simulink model "TST_CoETS_TrqCalc"  (R2016b)
settings: Solver=FixedStepDiscrete  StartTime=0.0  StopTime=simTime  FixedStep=sampleTime  RelTol=1e-3
values from neighbouring files (symbols this model uses):
  testCase = 1    [initTST_CoETS_TrqCalc_001.m]    (also in initTST_CoETS_TrqCalc_002.m = 2; initTST_CoETS_TrqCalc_003.m = 3)
libraries: simulink x52, UnitTest_Lib x48
(part 2 of 2)

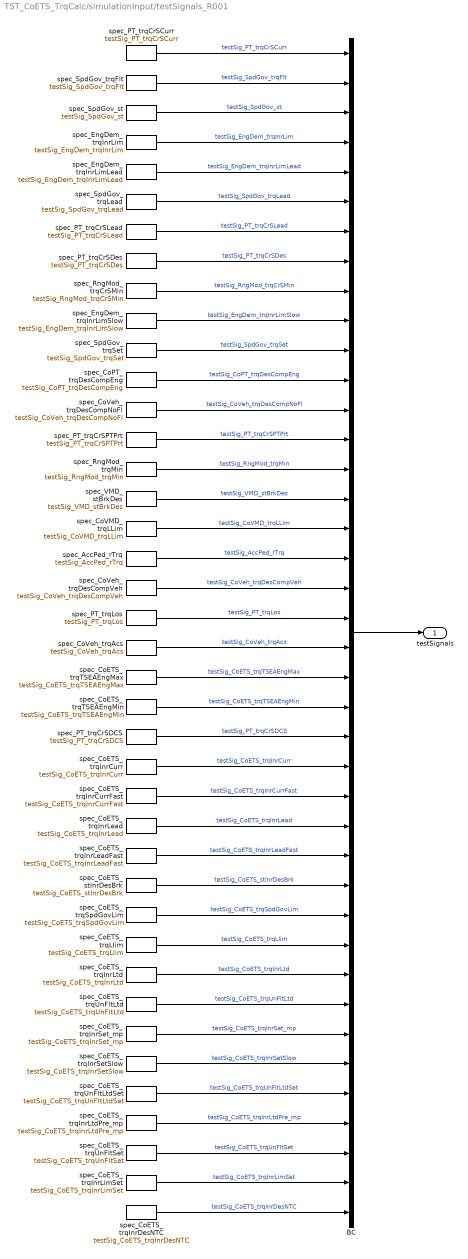
== system TST_CoETS_TrqCalc/simulationInput/testSignals_R001 ==
  BC : BusCreator  Inputs=40
  spec_AccPed_rTrq : FromWorkspace  VariableName=testSig_AccPed_rTrq  Interpolate=off  OutputAfterFinalValue=Holding final value
  spec_CoETS_stInrDesBrk : FromWorkspace  VariableName=testSig_CoETS_stInrDesBrk  Interpolate=off  OutputAfterFinalValue=Holding final value
  spec_CoETS_trqInrCurr : FromWorkspace  VariableName=testSig_CoETS_trqInrCurr  Interpolate=off  OutputAfterFinalValue=Holding final value
  spec_CoETS_trqInrCurrFast : FromWorkspace  VariableName=testSig_CoETS_trqInrCurrFast  Interpolate=off  OutputAfterFinalValue=Holding final value
  spec_CoETS_trqInrDesNTC : FromWorkspace  VariableName=testSig_CoETS_trqInrDesNTC  Interpolate=off  OutputAfterFinalValue=Holding final value
  spec_CoETS_trqInrLead : FromWorkspace  VariableName=testSig_CoETS_trqInrLead  Interpolate=off  OutputAfterFinalValue=Holding final value
  spec_CoETS_trqInrLeadFast : FromWorkspace  VariableName=testSig_CoETS_trqInrLeadFast  Interpolate=off  OutputAfterFinalValue=Holding final value
  spec_CoETS_trqInrLimSet : FromWorkspace  VariableName=testSig_CoETS_trqInrLimSet  Interpolate=off  OutputAfterFinalValue=Holding final value
  spec_CoETS_trqInrLtd : FromWorkspace  VariableName=testSig_CoETS_trqInrLtd  Interpolate=off  OutputAfterFinalValue=Holding final value
  spec_CoETS_trqInrLtdPre_mp : FromWorkspace  VariableName=testSig_CoETS_trqInrLtdPre_mp  Interpolate=off  OutputAfterFinalValue=Holding final value
  spec_CoETS_trqInrSetSlow : FromWorkspace  VariableName=testSig_CoETS_trqInrSetSlow  Interpolate=off  OutputAfterFinalValue=Holding final value
  spec_CoETS_trqInrSet_mp : FromWorkspace  VariableName=testSig_CoETS_trqInrSet_mp  Interpolate=off  OutputAfterFinalValue=Holding final value
  spec_CoETS_trqLlim : FromWorkspace  VariableName=testSig_CoETS_trqLlim  Interpolate=off  OutputAfterFinalValue=Holding final value
  spec_CoETS_trqSpdGovLim : FromWorkspace  VariableName=testSig_CoETS_trqSpdGovLim  Interpolate=off  OutputAfterFinalValue=Holding final value
  spec_CoETS_trqTSEAEngMax : FromWorkspace  VariableName=testSig_CoETS_trqTSEAEngMax  Interpolate=off  OutputAfterFinalValue=Holding final value
  spec_CoETS_trqTSEAEngMin : FromWorkspace  VariableName=testSig_CoETS_trqTSEAEngMin  Interpolate=off  OutputAfterFinalValue=Holding final value
  spec_CoETS_trqUnFltLtd : FromWorkspace  VariableName=testSig_CoETS_trqUnFltLtd  Interpolate=off  OutputAfterFinalValue=Holding final value
  spec_CoETS_trqUnFltLtdSet : FromWorkspace  VariableName=testSig_CoETS_trqUnFltLtdSet  Interpolate=off  OutputAfterFinalValue=Holding final value
  spec_CoETS_trqUnFltSet : FromWorkspace  VariableName=testSig_CoETS_trqUnFltSet  Interpolate=off  OutputAfterFinalValue=Holding final value
  spec_CoPT_trqDesCompEng : FromWorkspace  VariableName=testSig_CoPT_trqDesCompEng  Interpolate=off  OutputAfterFinalValue=Holding final value
  spec_CoVMD_trqLLim : FromWorkspace  VariableName=testSig_CoVMD_trqLLim  Interpolate=off  OutputAfterFinalValue=Holding final value
  spec_CoVeh_trqAcs : FromWorkspace  VariableName=testSig_CoVeh_trqAcs  Interpolate=off  OutputAfterFinalValue=Holding final value
  spec_CoVeh_trqDesCompNoFl : FromWorkspace  VariableName=testSig_CoVeh_trqDesCompNoFl  Interpolate=off  OutputAfterFinalValue=Holding final value
  spec_CoVeh_trqDesCompVeh : FromWorkspace  VariableName=testSig_CoVeh_trqDesCompVeh  Interpolate=off  OutputAfterFinalValue=Holding final value
  spec_EngDem_trqInrLim : FromWorkspace  VariableName=testSig_EngDem_trqInrLim  Interpolate=off  OutputAfterFinalValue=Holding final value
  spec_EngDem_trqInrLimLead : FromWorkspace  VariableName=testSig_EngDem_trqInrLimLead  Interpolate=off  OutputAfterFinalValue=Holding final value
  spec_EngDem_trqInrLimSlow : FromWorkspace  VariableName=testSig_EngDem_trqInrLimSlow  Interpolate=off  OutputAfterFinalValue=Holding final value
  spec_PT_trqCrSCurr : FromWorkspace  VariableName=testSig_PT_trqCrSCurr  Interpolate=off  OutputAfterFinalValue=Holding final value
  spec_PT_trqCrSDCS : FromWorkspace  VariableName=testSig_PT_trqCrSDCS  Interpolate=off  OutputAfterFinalValue=Holding final value
  spec_PT_trqCrSDes : FromWorkspace  VariableName=testSig_PT_trqCrSDes  Interpolate=off  OutputAfterFinalValue=Holding final value
  spec_PT_trqCrSLead : FromWorkspace  VariableName=testSig_PT_trqCrSLead  Interpolate=off  OutputAfterFinalValue=Holding final value
  spec_PT_trqCrSPTPrt : FromWorkspace  VariableName=testSig_PT_trqCrSPTPrt  Interpolate=off  OutputAfterFinalValue=Holding final value
  spec_PT_trqLos : FromWorkspace  VariableName=testSig_PT_trqLos  Interpolate=off  OutputAfterFinalValue=Holding final value
  spec_RngMod_trqCrSMin : FromWorkspace  VariableName=testSig_RngMod_trqCrSMin  Interpolate=off  OutputAfterFinalValue=Holding final value
  spec_RngMod_trqMin : FromWorkspace  VariableName=testSig_RngMod_trqMin  Interpolate=off  OutputAfterFinalValue=Holding final value
  spec_SpdGov_st : FromWorkspace  VariableName=testSig_SpdGov_st  Interpolate=off  OutputAfterFinalValue=Holding final value
  spec_SpdGov_trqFlt : FromWorkspace  VariableName=testSig_SpdGov_trqFlt  Interpolate=off  OutputAfterFinalValue=Holding final value
  spec_SpdGov_trqLead : FromWorkspace  VariableName=testSig_SpdGov_trqLead  Interpolate=off  OutputAfterFinalValue=Holding final value
  spec_SpdGov_trqSet : FromWorkspace  VariableName=testSig_SpdGov_trqSet  Interpolate=off  OutputAfterFinalValue=Holding final value
  spec_VMD_stBrkDes : FromWorkspace  VariableName=testSig_VMD_stBrkDes  Interpolate=off  OutputAfterFinalValue=Holding final value
  testSignals : Outport
  wires:
  BC/1 -> testSignals/1
  spec_PT_trqCrSCurr/1 -> BC/1  "testSig_PT_trqCrSCurr"
  spec_SpdGov_trqFlt/1 -> BC/2  "testSig_SpdGov_trqFlt"
  spec_SpdGov_st/1 -> BC/3  "testSig_SpdGov_st"
  spec_EngDem_trqInrLim/1 -> BC/4  "testSig_EngDem_trqInrLim"
  spec_EngDem_trqInrLimLead/1 -> BC/5  "testSig_EngDem_trqInrLimLead"
  spec_SpdGov_trqLead/1 -> BC/6  "testSig_SpdGov_trqLead"
  spec_PT_trqCrSLead/1 -> BC/7  "testSig_PT_trqCrSLead"
  spec_PT_trqCrSDes/1 -> BC/8  "testSig_PT_trqCrSDes"
  spec_RngMod_trqCrSMin/1 -> BC/9  "testSig_RngMod_trqCrSMin"
  spec_EngDem_trqInrLimSlow/1 -> BC/10  "testSig_EngDem_trqInrLimSlow"
  spec_SpdGov_trqSet/1 -> BC/11  "testSig_SpdGov_trqSet"
  spec_CoPT_trqDesCompEng/1 -> BC/12  "testSig_CoPT_trqDesCompEng"
  spec_CoVeh_trqDesCompNoFl/1 -> BC/13  "testSig_CoVeh_trqDesCompNoFl"
  spec_PT_trqCrSPTPrt/1 -> BC/14  "testSig_PT_trqCrSPTPrt"
  spec_RngMod_trqMin/1 -> BC/15  "testSig_RngMod_trqMin"
  spec_VMD_stBrkDes/1 -> BC/16  "testSig_VMD_stBrkDes"
  spec_CoVMD_trqLLim/1 -> BC/17  "testSig_CoVMD_trqLLim"
  spec_AccPed_rTrq/1 -> BC/18  "testSig_AccPed_rTrq"
  spec_CoVeh_trqDesCompVeh/1 -> BC/19  "testSig_CoVeh_trqDesCompVeh"
  spec_PT_trqLos/1 -> BC/20  "testSig_PT_trqLos"
  spec_CoVeh_trqAcs/1 -> BC/21  "testSig_CoVeh_trqAcs"
  spec_CoETS_trqTSEAEngMax/1 -> BC/22  "testSig_CoETS_trqTSEAEngMax"
  spec_CoETS_trqTSEAEngMin/1 -> BC/23  "testSig_CoETS_trqTSEAEngMin"
  spec_PT_trqCrSDCS/1 -> BC/24  "testSig_PT_trqCrSDCS"
  spec_CoETS_trqInrCurr/1 -> BC/25  "testSig_CoETS_trqInrCurr"
  spec_CoETS_trqInrCurrFast/1 -> BC/26  "testSig_CoETS_trqInrCurrFast"
  spec_CoETS_trqInrLead/1 -> BC/27  "testSig_CoETS_trqInrLead"
  spec_CoETS_trqInrLeadFast/1 -> BC/28  "testSig_CoETS_trqInrLeadFast"
  spec_CoETS_stInrDesBrk/1 -> BC/29  "testSig_CoETS_stInrDesBrk"
  spec_CoETS_trqSpdGovLim/1 -> BC/30  "testSig_CoETS_trqSpdGovLim"
  spec_CoETS_trqLlim/1 -> BC/31  "testSig_CoETS_trqLlim"
  spec_CoETS_trqInrLtd/1 -> BC/32  "testSig_CoETS_trqInrLtd"
  spec_CoETS_trqUnFltLtd/1 -> BC/33  "testSig_CoETS_trqUnFltLtd"
  spec_CoETS_trqInrSet_mp/1 -> BC/34  "testSig_CoETS_trqInrSet_mp"
  spec_CoETS_trqInrSetSlow/1 -> BC/35  "testSig_CoETS_trqInrSetSlow"
  spec_CoETS_trqUnFltLtdSet/1 -> BC/36  "testSig_CoETS_trqUnFltLtdSet"
  spec_CoETS_trqInrLtdPre_mp/1 -> BC/37  "testSig_CoETS_trqInrLtdPre_mp"
  spec_CoETS_trqUnFltSet/1 -> BC/38  "testSig_CoETS_trqUnFltSet"
  spec_CoETS_trqInrLimSet/1 -> BC/39  "testSig_CoETS_trqInrLimSet"
  spec_CoETS_trqInrDesNTC/1 -> BC/40  "testSig_CoETS_trqInrDesNTC"

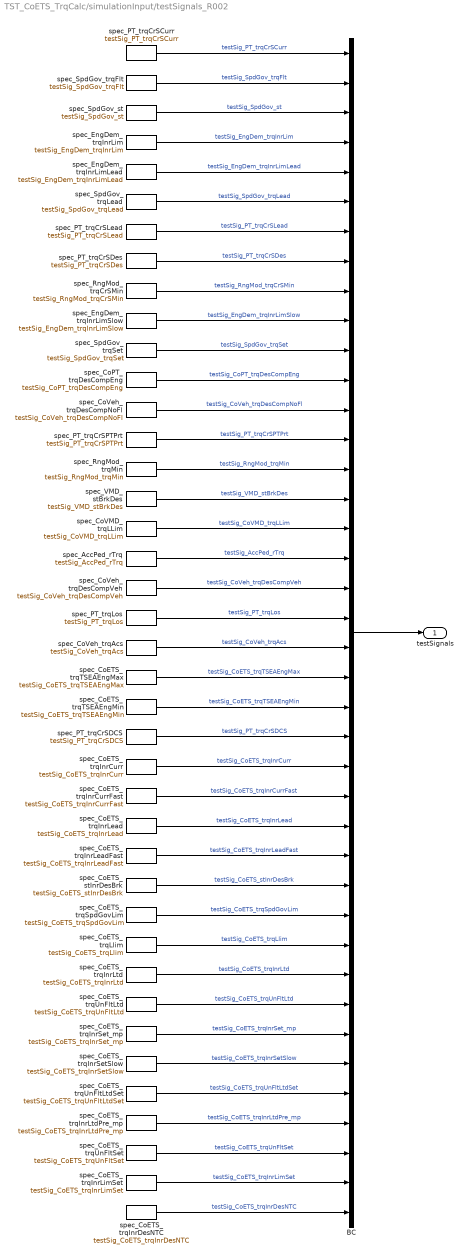
== system TST_CoETS_TrqCalc/simulationInput/testSignals_R002 ==
  BC : BusCreator  Inputs=40
  spec_AccPed_rTrq : FromWorkspace  VariableName=testSig_AccPed_rTrq  Interpolate=off  OutputAfterFinalValue=Holding final value
  spec_CoETS_stInrDesBrk : FromWorkspace  VariableName=testSig_CoETS_stInrDesBrk  Interpolate=off  OutputAfterFinalValue=Holding final value
  spec_CoETS_trqInrCurr : FromWorkspace  VariableName=testSig_CoETS_trqInrCurr  Interpolate=off  OutputAfterFinalValue=Holding final value
  spec_CoETS_trqInrCurrFast : FromWorkspace  VariableName=testSig_CoETS_trqInrCurrFast  Interpolate=off  OutputAfterFinalValue=Holding final value
  spec_CoETS_trqInrDesNTC : FromWorkspace  VariableName=testSig_CoETS_trqInrDesNTC  Interpolate=off  OutputAfterFinalValue=Holding final value
  spec_CoETS_trqInrLead : FromWorkspace  VariableName=testSig_CoETS_trqInrLead  Interpolate=off  OutputAfterFinalValue=Holding final value
  spec_CoETS_trqInrLeadFast : FromWorkspace  VariableName=testSig_CoETS_trqInrLeadFast  Interpolate=off  OutputAfterFinalValue=Holding final value
  spec_CoETS_trqInrLimSet : FromWorkspace  VariableName=testSig_CoETS_trqInrLimSet  Interpolate=off  OutputAfterFinalValue=Holding final value
  spec_CoETS_trqInrLtd : FromWorkspace  VariableName=testSig_CoETS_trqInrLtd  Interpolate=off  OutputAfterFinalValue=Holding final value
  spec_CoETS_trqInrLtdPre_mp : FromWorkspace  VariableName=testSig_CoETS_trqInrLtdPre_mp  Interpolate=off  OutputAfterFinalValue=Holding final value
  spec_CoETS_trqInrSetSlow : FromWorkspace  VariableName=testSig_CoETS_trqInrSetSlow  Interpolate=off  OutputAfterFinalValue=Holding final value
  spec_CoETS_trqInrSet_mp : FromWorkspace  VariableName=testSig_CoETS_trqInrSet_mp  Interpolate=off  OutputAfterFinalValue=Holding final value
  spec_CoETS_trqLlim : FromWorkspace  VariableName=testSig_CoETS_trqLlim  Interpolate=off  OutputAfterFinalValue=Holding final value
  spec_CoETS_trqSpdGovLim : FromWorkspace  VariableName=testSig_CoETS_trqSpdGovLim  Interpolate=off  OutputAfterFinalValue=Holding final value
  spec_CoETS_trqTSEAEngMax : FromWorkspace  VariableName=testSig_CoETS_trqTSEAEngMax  Interpolate=off  OutputAfterFinalValue=Holding final value
  spec_CoETS_trqTSEAEngMin : FromWorkspace  VariableName=testSig_CoETS_trqTSEAEngMin  Interpolate=off  OutputAfterFinalValue=Holding final value
  spec_CoETS_trqUnFltLtd : FromWorkspace  VariableName=testSig_CoETS_trqUnFltLtd  Interpolate=off  OutputAfterFinalValue=Holding final value
  spec_CoETS_trqUnFltLtdSet : FromWorkspace  VariableName=testSig_CoETS_trqUnFltLtdSet  Interpolate=off  OutputAfterFinalValue=Holding final value
  spec_CoETS_trqUnFltSet : FromWorkspace  VariableName=testSig_CoETS_trqUnFltSet  Interpolate=off  OutputAfterFinalValue=Holding final value
  spec_CoPT_trqDesCompEng : FromWorkspace  VariableName=testSig_CoPT_trqDesCompEng  Interpolate=off  OutputAfterFinalValue=Holding final value
  spec_CoVMD_trqLLim : FromWorkspace  VariableName=testSig_CoVMD_trqLLim  Interpolate=off  OutputAfterFinalValue=Holding final value
  spec_CoVeh_trqAcs : FromWorkspace  VariableName=testSig_CoVeh_trqAcs  Interpolate=off  OutputAfterFinalValue=Holding final value
  spec_CoVeh_trqDesCompNoFl : FromWorkspace  VariableName=testSig_CoVeh_trqDesCompNoFl  Interpolate=off  OutputAfterFinalValue=Holding final value
  spec_CoVeh_trqDesCompVeh : FromWorkspace  VariableName=testSig_CoVeh_trqDesCompVeh  Interpolate=off  OutputAfterFinalValue=Holding final value
  spec_EngDem_trqInrLim : FromWorkspace  VariableName=testSig_EngDem_trqInrLim  Interpolate=off  OutputAfterFinalValue=Holding final value
  spec_EngDem_trqInrLimLead : FromWorkspace  VariableName=testSig_EngDem_trqInrLimLead  Interpolate=off  OutputAfterFinalValue=Holding final value
  spec_EngDem_trqInrLimSlow : FromWorkspace  VariableName=testSig_EngDem_trqInrLimSlow  Interpolate=off  OutputAfterFinalValue=Holding final value
  spec_PT_trqCrSCurr : FromWorkspace  VariableName=testSig_PT_trqCrSCurr  Interpolate=off  OutputAfterFinalValue=Holding final value
  spec_PT_trqCrSDCS : FromWorkspace  VariableName=testSig_PT_trqCrSDCS  Interpolate=off  OutputAfterFinalValue=Holding final value
  spec_PT_trqCrSDes : FromWorkspace  VariableName=testSig_PT_trqCrSDes  Interpolate=off  OutputAfterFinalValue=Holding final value
  spec_PT_trqCrSLead : FromWorkspace  VariableName=testSig_PT_trqCrSLead  Interpolate=off  OutputAfterFinalValue=Holding final value
  spec_PT_trqCrSPTPrt : FromWorkspace  VariableName=testSig_PT_trqCrSPTPrt  Interpolate=off  OutputAfterFinalValue=Holding final value
  spec_PT_trqLos : FromWorkspace  VariableName=testSig_PT_trqLos  Interpolate=off  OutputAfterFinalValue=Holding final value
  spec_RngMod_trqCrSMin : FromWorkspace  VariableName=testSig_RngMod_trqCrSMin  Interpolate=off  OutputAfterFinalValue=Holding final value
  spec_RngMod_trqMin : FromWorkspace  VariableName=testSig_RngMod_trqMin  Interpolate=off  OutputAfterFinalValue=Holding final value
  spec_SpdGov_st : FromWorkspace  VariableName=testSig_SpdGov_st  Interpolate=off  OutputAfterFinalValue=Holding final value
  spec_SpdGov_trqFlt : FromWorkspace  VariableName=testSig_SpdGov_trqFlt  Interpolate=off  OutputAfterFinalValue=Holding final value
  spec_SpdGov_trqLead : FromWorkspace  VariableName=testSig_SpdGov_trqLead  Interpolate=off  OutputAfterFinalValue=Holding final value
  spec_SpdGov_trqSet : FromWorkspace  VariableName=testSig_SpdGov_trqSet  Interpolate=off  OutputAfterFinalValue=Holding final value
  spec_VMD_stBrkDes : FromWorkspace  VariableName=testSig_VMD_stBrkDes  Interpolate=off  OutputAfterFinalValue=Holding final value
  testSignals : Outport
  wires:
  BC/1 -> testSignals/1
  spec_PT_trqCrSCurr/1 -> BC/1  "testSig_PT_trqCrSCurr"
  spec_SpdGov_trqFlt/1 -> BC/2  "testSig_SpdGov_trqFlt"
  spec_SpdGov_st/1 -> BC/3  "testSig_SpdGov_st"
  spec_EngDem_trqInrLim/1 -> BC/4  "testSig_EngDem_trqInrLim"
  spec_EngDem_trqInrLimLead/1 -> BC/5  "testSig_EngDem_trqInrLimLead"
  spec_SpdGov_trqLead/1 -> BC/6  "testSig_SpdGov_trqLead"
  spec_PT_trqCrSLead/1 -> BC/7  "testSig_PT_trqCrSLead"
  spec_PT_trqCrSDes/1 -> BC/8  "testSig_PT_trqCrSDes"
  spec_RngMod_trqCrSMin/1 -> BC/9  "testSig_RngMod_trqCrSMin"
  spec_EngDem_trqInrLimSlow/1 -> BC/10  "testSig_EngDem_trqInrLimSlow"
  spec_SpdGov_trqSet/1 -> BC/11  "testSig_SpdGov_trqSet"
  spec_CoPT_trqDesCompEng/1 -> BC/12  "testSig_CoPT_trqDesCompEng"
  spec_CoVeh_trqDesCompNoFl/1 -> BC/13  "testSig_CoVeh_trqDesCompNoFl"
  spec_PT_trqCrSPTPrt/1 -> BC/14  "testSig_PT_trqCrSPTPrt"
  spec_RngMod_trqMin/1 -> BC/15  "testSig_RngMod_trqMin"
  spec_VMD_stBrkDes/1 -> BC/16  "testSig_VMD_stBrkDes"
  spec_CoVMD_trqLLim/1 -> BC/17  "testSig_CoVMD_trqLLim"
  spec_AccPed_rTrq/1 -> BC/18  "testSig_AccPed_rTrq"
  spec_CoVeh_trqDesCompVeh/1 -> BC/19  "testSig_CoVeh_trqDesCompVeh"
  spec_PT_trqLos/1 -> BC/20  "testSig_PT_trqLos"
  spec_CoVeh_trqAcs/1 -> BC/21  "testSig_CoVeh_trqAcs"
  spec_CoETS_trqTSEAEngMax/1 -> BC/22  "testSig_CoETS_trqTSEAEngMax"
  spec_CoETS_trqTSEAEngMin/1 -> BC/23  "testSig_CoETS_trqTSEAEngMin"
  spec_PT_trqCrSDCS/1 -> BC/24  "testSig_PT_trqCrSDCS"
  spec_CoETS_trqInrCurr/1 -> BC/25  "testSig_CoETS_trqInrCurr"
  spec_CoETS_trqInrCurrFast/1 -> BC/26  "testSig_CoETS_trqInrCurrFast"
  spec_CoETS_trqInrLead/1 -> BC/27  "testSig_CoETS_trqInrLead"
  spec_CoETS_trqInrLeadFast/1 -> BC/28  "testSig_CoETS_trqInrLeadFast"
  spec_CoETS_stInrDesBrk/1 -> BC/29  "testSig_CoETS_stInrDesBrk"
  spec_CoETS_trqSpdGovLim/1 -> BC/30  "testSig_CoETS_trqSpdGovLim"
  spec_CoETS_trqLlim/1 -> BC/31  "testSig_CoETS_trqLlim"
  spec_CoETS_trqInrLtd/1 -> BC/32  "testSig_CoETS_trqInrLtd"
  spec_CoETS_trqUnFltLtd/1 -> BC/33  "testSig_CoETS_trqUnFltLtd"
  spec_CoETS_trqInrSet_mp/1 -> BC/34  "testSig_CoETS_trqInrSet_mp"
  spec_CoETS_trqInrSetSlow/1 -> BC/35  "testSig_CoETS_trqInrSetSlow"
  spec_CoETS_trqUnFltLtdSet/1 -> BC/36  "testSig_CoETS_trqUnFltLtdSet"
  spec_CoETS_trqInrLtdPre_mp/1 -> BC/37  "testSig_CoETS_trqInrLtdPre_mp"
  spec_CoETS_trqUnFltSet/1 -> BC/38  "testSig_CoETS_trqUnFltSet"
  spec_CoETS_trqInrLimSet/1 -> BC/39  "testSig_CoETS_trqInrLimSet"
  spec_CoETS_trqInrDesNTC/1 -> BC/40  "testSig_CoETS_trqInrDesNTC"

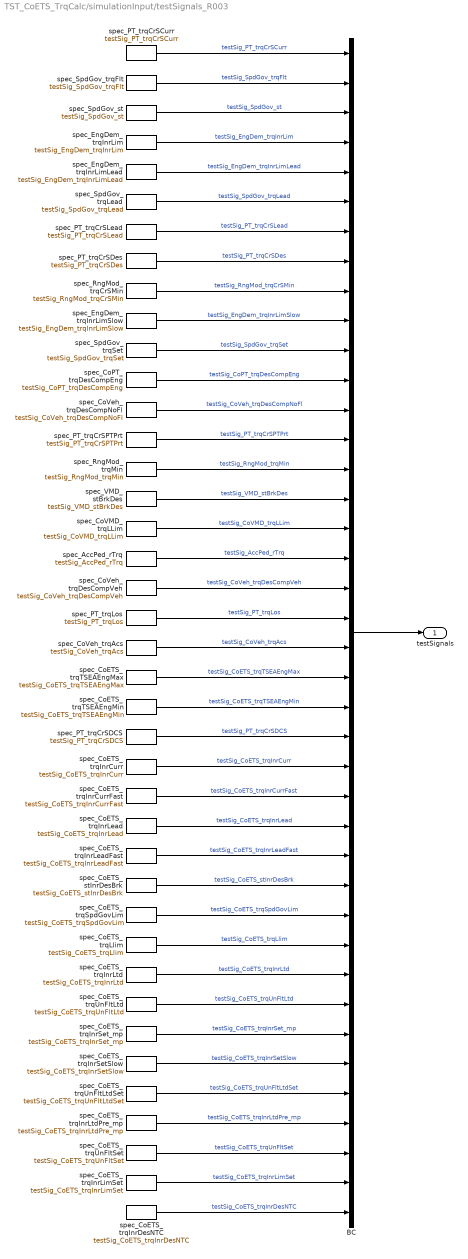
== system TST_CoETS_TrqCalc/simulationInput/testSignals_R003 ==
  BC : BusCreator  Inputs=40
  spec_AccPed_rTrq : FromWorkspace  VariableName=testSig_AccPed_rTrq  Interpolate=off  OutputAfterFinalValue=Holding final value
  spec_CoETS_stInrDesBrk : FromWorkspace  VariableName=testSig_CoETS_stInrDesBrk  Interpolate=off  OutputAfterFinalValue=Holding final value
  spec_CoETS_trqInrCurr : FromWorkspace  VariableName=testSig_CoETS_trqInrCurr  Interpolate=off  OutputAfterFinalValue=Holding final value
  spec_CoETS_trqInrCurrFast : FromWorkspace  VariableName=testSig_CoETS_trqInrCurrFast  Interpolate=off  OutputAfterFinalValue=Holding final value
  spec_CoETS_trqInrDesNTC : FromWorkspace  VariableName=testSig_CoETS_trqInrDesNTC  Interpolate=off  OutputAfterFinalValue=Holding final value
  spec_CoETS_trqInrLead : FromWorkspace  VariableName=testSig_CoETS_trqInrLead  Interpolate=off  OutputAfterFinalValue=Holding final value
  spec_CoETS_trqInrLeadFast : FromWorkspace  VariableName=testSig_CoETS_trqInrLeadFast  Interpolate=off  OutputAfterFinalValue=Holding final value
  spec_CoETS_trqInrLimSet : FromWorkspace  VariableName=testSig_CoETS_trqInrLimSet  Interpolate=off  OutputAfterFinalValue=Holding final value
  spec_CoETS_trqInrLtd : FromWorkspace  VariableName=testSig_CoETS_trqInrLtd  Interpolate=off  OutputAfterFinalValue=Holding final value
  spec_CoETS_trqInrLtdPre_mp : FromWorkspace  VariableName=testSig_CoETS_trqInrLtdPre_mp  Interpolate=off  OutputAfterFinalValue=Holding final value
  spec_CoETS_trqInrSetSlow : FromWorkspace  VariableName=testSig_CoETS_trqInrSetSlow  Interpolate=off  OutputAfterFinalValue=Holding final value
  spec_CoETS_trqInrSet_mp : FromWorkspace  VariableName=testSig_CoETS_trqInrSet_mp  Interpolate=off  OutputAfterFinalValue=Holding final value
  spec_CoETS_trqLlim : FromWorkspace  VariableName=testSig_CoETS_trqLlim  Interpolate=off  OutputAfterFinalValue=Holding final value
  spec_CoETS_trqSpdGovLim : FromWorkspace  VariableName=testSig_CoETS_trqSpdGovLim  Interpolate=off  OutputAfterFinalValue=Holding final value
  spec_CoETS_trqTSEAEngMax : FromWorkspace  VariableName=testSig_CoETS_trqTSEAEngMax  Interpolate=off  OutputAfterFinalValue=Holding final value
  spec_CoETS_trqTSEAEngMin : FromWorkspace  VariableName=testSig_CoETS_trqTSEAEngMin  Interpolate=off  OutputAfterFinalValue=Holding final value
  spec_CoETS_trqUnFltLtd : FromWorkspace  VariableName=testSig_CoETS_trqUnFltLtd  Interpolate=off  OutputAfterFinalValue=Holding final value
  spec_CoETS_trqUnFltLtdSet : FromWorkspace  VariableName=testSig_CoETS_trqUnFltLtdSet  Interpolate=off  OutputAfterFinalValue=Holding final value
  spec_CoETS_trqUnFltSet : FromWorkspace  VariableName=testSig_CoETS_trqUnFltSet  Interpolate=off  OutputAfterFinalValue=Holding final value
  spec_CoPT_trqDesCompEng : FromWorkspace  VariableName=testSig_CoPT_trqDesCompEng  Interpolate=off  OutputAfterFinalValue=Holding final value
  spec_CoVMD_trqLLim : FromWorkspace  VariableName=testSig_CoVMD_trqLLim  Interpolate=off  OutputAfterFinalValue=Holding final value
  spec_CoVeh_trqAcs : FromWorkspace  VariableName=testSig_CoVeh_trqAcs  Interpolate=off  OutputAfterFinalValue=Holding final value
  spec_CoVeh_trqDesCompNoFl : FromWorkspace  VariableName=testSig_CoVeh_trqDesCompNoFl  Interpolate=off  OutputAfterFinalValue=Holding final value
  spec_CoVeh_trqDesCompVeh : FromWorkspace  VariableName=testSig_CoVeh_trqDesCompVeh  Interpolate=off  OutputAfterFinalValue=Holding final value
  spec_EngDem_trqInrLim : FromWorkspace  VariableName=testSig_EngDem_trqInrLim  Interpolate=off  OutputAfterFinalValue=Holding final value
  spec_EngDem_trqInrLimLead : FromWorkspace  VariableName=testSig_EngDem_trqInrLimLead  Interpolate=off  OutputAfterFinalValue=Holding final value
  spec_EngDem_trqInrLimSlow : FromWorkspace  VariableName=testSig_EngDem_trqInrLimSlow  Interpolate=off  OutputAfterFinalValue=Holding final value
  spec_PT_trqCrSCurr : FromWorkspace  VariableName=testSig_PT_trqCrSCurr  Interpolate=off  OutputAfterFinalValue=Holding final value
  spec_PT_trqCrSDCS : FromWorkspace  VariableName=testSig_PT_trqCrSDCS  Interpolate=off  OutputAfterFinalValue=Holding final value
  spec_PT_trqCrSDes : FromWorkspace  VariableName=testSig_PT_trqCrSDes  Interpolate=off  OutputAfterFinalValue=Holding final value
  spec_PT_trqCrSLead : FromWorkspace  VariableName=testSig_PT_trqCrSLead  Interpolate=off  OutputAfterFinalValue=Holding final value
  spec_PT_trqCrSPTPrt : FromWorkspace  VariableName=testSig_PT_trqCrSPTPrt  Interpolate=off  OutputAfterFinalValue=Holding final value
  spec_PT_trqLos : FromWorkspace  VariableName=testSig_PT_trqLos  Interpolate=off  OutputAfterFinalValue=Holding final value
  spec_RngMod_trqCrSMin : FromWorkspace  VariableName=testSig_RngMod_trqCrSMin  Interpolate=off  OutputAfterFinalValue=Holding final value
  spec_RngMod_trqMin : FromWorkspace  VariableName=testSig_RngMod_trqMin  Interpolate=off  OutputAfterFinalValue=Holding final value
  spec_SpdGov_st : FromWorkspace  VariableName=testSig_SpdGov_st  Interpolate=off  OutputAfterFinalValue=Holding final value
  spec_SpdGov_trqFlt : FromWorkspace  VariableName=testSig_SpdGov_trqFlt  Interpolate=off  OutputAfterFinalValue=Holding final value
  spec_SpdGov_trqLead : FromWorkspace  VariableName=testSig_SpdGov_trqLead  Interpolate=off  OutputAfterFinalValue=Holding final value
  spec_SpdGov_trqSet : FromWorkspace  VariableName=testSig_SpdGov_trqSet  Interpolate=off  OutputAfterFinalValue=Holding final value
  spec_VMD_stBrkDes : FromWorkspace  VariableName=testSig_VMD_stBrkDes  Interpolate=off  OutputAfterFinalValue=Holding final value
  testSignals : Outport
  wires:
  BC/1 -> testSignals/1
  spec_PT_trqCrSCurr/1 -> BC/1  "testSig_PT_trqCrSCurr"
  spec_SpdGov_trqFlt/1 -> BC/2  "testSig_SpdGov_trqFlt"
  spec_SpdGov_st/1 -> BC/3  "testSig_SpdGov_st"
  spec_EngDem_trqInrLim/1 -> BC/4  "testSig_EngDem_trqInrLim"
  spec_EngDem_trqInrLimLead/1 -> BC/5  "testSig_EngDem_trqInrLimLead"
  spec_SpdGov_trqLead/1 -> BC/6  "testSig_SpdGov_trqLead"
  spec_PT_trqCrSLead/1 -> BC/7  "testSig_PT_trqCrSLead"
  spec_PT_trqCrSDes/1 -> BC/8  "testSig_PT_trqCrSDes"
  spec_RngMod_trqCrSMin/1 -> BC/9  "testSig_RngMod_trqCrSMin"
  spec_EngDem_trqInrLimSlow/1 -> BC/10  "testSig_EngDem_trqInrLimSlow"
  spec_SpdGov_trqSet/1 -> BC/11  "testSig_SpdGov_trqSet"
  spec_CoPT_trqDesCompEng/1 -> BC/12  "testSig_CoPT_trqDesCompEng"
  spec_CoVeh_trqDesCompNoFl/1 -> BC/13  "testSig_CoVeh_trqDesCompNoFl"
  spec_PT_trqCrSPTPrt/1 -> BC/14  "testSig_PT_trqCrSPTPrt"
  spec_RngMod_trqMin/1 -> BC/15  "testSig_RngMod_trqMin"
  spec_VMD_stBrkDes/1 -> BC/16  "testSig_VMD_stBrkDes"
  spec_CoVMD_trqLLim/1 -> BC/17  "testSig_CoVMD_trqLLim"
  spec_AccPed_rTrq/1 -> BC/18  "testSig_AccPed_rTrq"
  spec_CoVeh_trqDesCompVeh/1 -> BC/19  "testSig_CoVeh_trqDesCompVeh"
  spec_PT_trqLos/1 -> BC/20  "testSig_PT_trqLos"
  spec_CoVeh_trqAcs/1 -> BC/21  "testSig_CoVeh_trqAcs"
  spec_CoETS_trqTSEAEngMax/1 -> BC/22  "testSig_CoETS_trqTSEAEngMax"
  spec_CoETS_trqTSEAEngMin/1 -> BC/23  "testSig_CoETS_trqTSEAEngMin"
  spec_PT_trqCrSDCS/1 -> BC/24  "testSig_PT_trqCrSDCS"
  spec_CoETS_trqInrCurr/1 -> BC/25  "testSig_CoETS_trqInrCurr"
  spec_CoETS_trqInrCurrFast/1 -> BC/26  "testSig_CoETS_trqInrCurrFast"
  spec_CoETS_trqInrLead/1 -> BC/27  "testSig_CoETS_trqInrLead"
  spec_CoETS_trqInrLeadFast/1 -> BC/28  "testSig_CoETS_trqInrLeadFast"
  spec_CoETS_stInrDesBrk/1 -> BC/29  "testSig_CoETS_stInrDesBrk"
  spec_CoETS_trqSpdGovLim/1 -> BC/30  "testSig_CoETS_trqSpdGovLim"
  spec_CoETS_trqLlim/1 -> BC/31  "testSig_CoETS_trqLlim"
  spec_CoETS_trqInrLtd/1 -> BC/32  "testSig_CoETS_trqInrLtd"
  spec_CoETS_trqUnFltLtd/1 -> BC/33  "testSig_CoETS_trqUnFltLtd"
  spec_CoETS_trqInrSet_mp/1 -> BC/34  "testSig_CoETS_trqInrSet_mp"
  spec_CoETS_trqInrSetSlow/1 -> BC/35  "testSig_CoETS_trqInrSetSlow"
  spec_CoETS_trqUnFltLtdSet/1 -> BC/36  "testSig_CoETS_trqUnFltLtdSet"
  spec_CoETS_trqInrLtdPre_mp/1 -> BC/37  "testSig_CoETS_trqInrLtdPre_mp"
  spec_CoETS_trqUnFltSet/1 -> BC/38  "testSig_CoETS_trqUnFltSet"
  spec_CoETS_trqInrLimSet/1 -> BC/39  "testSig_CoETS_trqInrLimSet"
  spec_CoETS_trqInrDesNTC/1 -> BC/40  "testSig_CoETS_trqInrDesNTC"

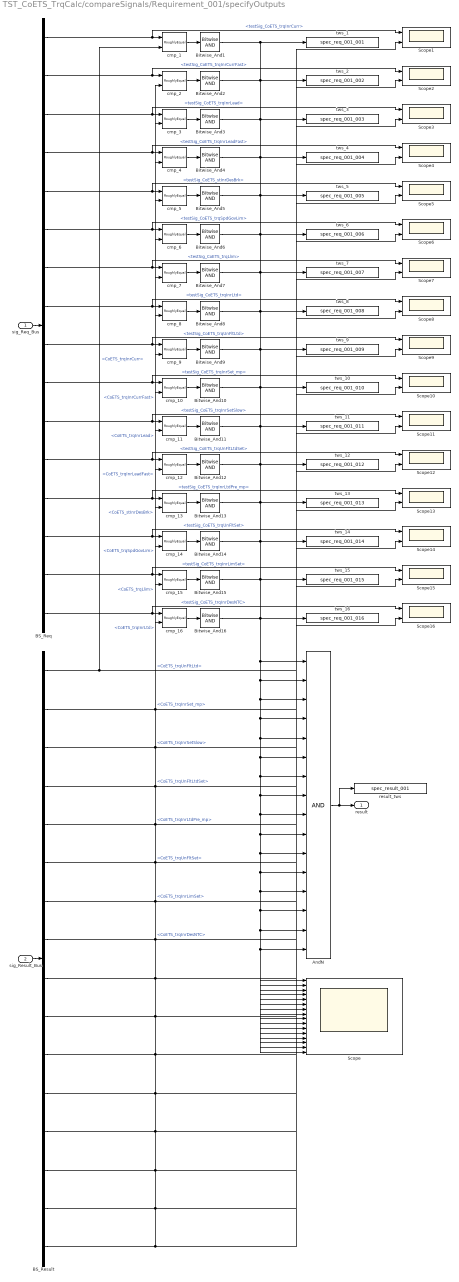
== system TST_CoETS_TrqCalc/compareSignals/Requirement_001/specifyOutputs ==
  sig_Req_Bus : Inport
  sig_Result_Bus : Inport  Port=2
  AndN : Logic  Inputs=16
  BS_Req : BusSelector  OutputSignals=testSig_CoETS_trqInrCurr,testSig_CoETS_trqInrCurrFast,testSig_CoETS_trqInrLead,testSig_CoETS_trqInrLeadFast,testSig_CoETS_stInrDesBrk,testSig_CoETS_trqSpdGovLim,testSig_CoETS_trqLlim,testSig_CoETS_trqInrLtd,testSig_CoETS_trqUnFltLtd,testSig_CoETS_trqInrSet_mp,testSig_CoETS_trqInrSetSlow,testSig_CoETS_trqUnFltLtdSet,testSig_CoETS_trqInrLtdPre_mp,testSig_CoETS_trqUnFltSet,testSig_CoETS_trqInrLimSet,testSig_CoETS_trqInrDesNTC
  BS_Result : BusSelector  OutputSignals=CoETS_trqInrCurr,CoETS_trqInrCurrFast,CoETS_trqInrLead,CoETS_trqInrLeadFast,CoETS_stInrDesBrk,CoETS_trqSpdGovLim,CoETS_trqLlim,CoETS_trqInrLtd,CoETS_trqUnFltLtd,CoETS_trqInrSet_mp,CoETS_trqInrSetSlow,CoETS_trqUnFltLtdSet,CoETS_trqInrLtdPre_mp,CoETS_trqUnFltSet,CoETS_trqInrLimSet,CoETS_trqInrDesNTC
  Bitwise_And{1..16} (16 alike) : simulink/Logic and Bit Operations/Bitwise Operator  logicop=AND  UseBitMask=off  BitMask=bin2dec('11011001')  BitMaskRealWorld=Stored Integer
  Scope : Scope  NumInputPorts=16
  Scope{1..16} (16 alike) : Scope  NumInputPorts=2
  cmp_{1,3..16} (15 alike) : UnitTest_Lib/RoughlyEqual  slope=0.1
  cmp_2 : UnitTest_Lib/RoughlyEqual  slope=0.5
  result_tws : ToWorkspace  VariableName=spec_result_001
  tws_1 : ToWorkspace  VariableName=spec_req_001_001
  tws_10 : ToWorkspace  VariableName=spec_req_001_010
  tws_11 : ToWorkspace  VariableName=spec_req_001_011
  tws_12 : ToWorkspace  VariableName=spec_req_001_012
  tws_13 : ToWorkspace  VariableName=spec_req_001_013
  tws_14 : ToWorkspace  VariableName=spec_req_001_014
  tws_15 : ToWorkspace  VariableName=spec_req_001_015
  tws_16 : ToWorkspace  VariableName=spec_req_001_016
  tws_2 : ToWorkspace  VariableName=spec_req_001_002
  tws_3 : ToWorkspace  VariableName=spec_req_001_003
  tws_4 : ToWorkspace  VariableName=spec_req_001_004
  tws_5 : ToWorkspace  VariableName=spec_req_001_005
  tws_6 : ToWorkspace  VariableName=spec_req_001_006
  tws_7 : ToWorkspace  VariableName=spec_req_001_007
  tws_8 : ToWorkspace  VariableName=spec_req_001_008
  tws_9 : ToWorkspace  VariableName=spec_req_001_009
  result : Outport
  wires:
  sig_Req_Bus/1 -> BS_Req/1
  sig_Result_Bus/1 -> BS_Result/1
  AndN/1 -> result/1, result_tws/1
  BS_Req/1 -> cmp_1/1, Scope1/1  "<testSig_CoETS_trqInrCurr>"
  BS_Result/1 -> cmp_1/2, Scope1/2  "<CoETS_trqInrCurr>"
  cmp_1/1 -> Bitwise_And1/1
  Bitwise_And1/1 -> AndN/1, Scope/1, tws_1/1
  BS_Req/2 -> cmp_2/1, Scope2/1  "<testSig_CoETS_trqInrCurrFast>"
  BS_Result/2 -> cmp_2/2, Scope2/2  "<CoETS_trqInrCurrFast>"
  cmp_2/1 -> Bitwise_And2/1
  Bitwise_And2/1 -> AndN/2, Scope/2, tws_2/1
  BS_Req/3 -> cmp_3/1, Scope3/1  "<testSig_CoETS_trqInrLead>"
  BS_Result/3 -> cmp_3/2, Scope3/2  "<CoETS_trqInrLead>"
  cmp_3/1 -> Bitwise_And3/1
  Bitwise_And3/1 -> AndN/3, Scope/3, tws_3/1
  BS_Req/4 -> cmp_4/1, Scope4/1  "<testSig_CoETS_trqInrLeadFast>"
  BS_Result/4 -> cmp_4/2, Scope4/2  "<CoETS_trqInrLeadFast>"
  cmp_4/1 -> Bitwise_And4/1
  Bitwise_And4/1 -> AndN/4, Scope/4, tws_4/1
  BS_Req/5 -> cmp_5/1, Scope5/1  "<testSig_CoETS_stInrDesBrk>"
  BS_Result/5 -> cmp_5/2, Scope5/2  "<CoETS_stInrDesBrk>"
  cmp_5/1 -> Bitwise_And5/1
  Bitwise_And5/1 -> AndN/5, Scope/5, tws_5/1
  BS_Req/6 -> cmp_6/1, Scope6/1  "<testSig_CoETS_trqSpdGovLim>"
  BS_Result/6 -> cmp_6/2, Scope6/2  "<CoETS_trqSpdGovLim>"
  cmp_6/1 -> Bitwise_And6/1
  Bitwise_And6/1 -> AndN/6, Scope/6, tws_6/1
  BS_Req/7 -> cmp_7/1, Scope7/1  "<testSig_CoETS_trqLlim>"
  BS_Result/7 -> cmp_7/2, Scope7/2  "<CoETS_trqLlim>"
  cmp_7/1 -> Bitwise_And7/1
  Bitwise_And7/1 -> AndN/7, Scope/7, tws_7/1
  BS_Req/8 -> cmp_8/1, Scope8/1  "<testSig_CoETS_trqInrLtd>"
  BS_Result/8 -> cmp_8/2, Scope8/2  "<CoETS_trqInrLtd>"
  cmp_8/1 -> Bitwise_And8/1
  Bitwise_And8/1 -> AndN/8, Scope/8, tws_8/1
  BS_Req/9 -> cmp_9/1, Scope9/1  "<testSig_CoETS_trqUnFltLtd>"
  BS_Result/9 -> cmp_9/2, Scope9/2  "<CoETS_trqUnFltLtd>"
  cmp_9/1 -> Bitwise_And9/1
  Bitwise_And9/1 -> AndN/9, Scope/9, tws_9/1
  BS_Req/10 -> cmp_10/1, Scope10/1  "<testSig_CoETS_trqInrSet_mp>"
  BS_Result/10 -> cmp_10/2, Scope10/2  "<CoETS_trqInrSet_mp>"
  cmp_10/1 -> Bitwise_And10/1
  Bitwise_And10/1 -> AndN/10, Scope/10, tws_10/1
  BS_Req/11 -> cmp_11/1, Scope11/1  "<testSig_CoETS_trqInrSetSlow>"
  BS_Result/11 -> cmp_11/2, Scope11/2  "<CoETS_trqInrSetSlow>"
  cmp_11/1 -> Bitwise_And11/1
  Bitwise_And11/1 -> AndN/11, Scope/11, tws_11/1
  BS_Req/12 -> cmp_12/1, Scope12/1  "<testSig_CoETS_trqUnFltLtdSet>"
  BS_Result/12 -> cmp_12/2, Scope12/2  "<CoETS_trqUnFltLtdSet>"
  cmp_12/1 -> Bitwise_And12/1
  Bitwise_And12/1 -> AndN/12, Scope/12, tws_12/1
  BS_Req/13 -> cmp_13/1, Scope13/1  "<testSig_CoETS_trqInrLtdPre_mp>"
  BS_Result/13 -> cmp_13/2, Scope13/2  "<CoETS_trqInrLtdPre_mp>"
  cmp_13/1 -> Bitwise_And13/1
  Bitwise_And13/1 -> AndN/13, Scope/13, tws_13/1
  BS_Req/14 -> cmp_14/1, Scope14/1  "<testSig_CoETS_trqUnFltSet>"
  BS_Result/14 -> cmp_14/2, Scope14/2  "<CoETS_trqUnFltSet>"
  cmp_14/1 -> Bitwise_And14/1
  Bitwise_And14/1 -> AndN/14, Scope/14, tws_14/1
  BS_Req/15 -> cmp_15/1, Scope15/1  "<testSig_CoETS_trqInrLimSet>"
  BS_Result/15 -> cmp_15/2, Scope15/2  "<CoETS_trqInrLimSet>"
  cmp_15/1 -> Bitwise_And15/1
  Bitwise_And15/1 -> AndN/15, Scope/15, tws_15/1
  BS_Req/16 -> cmp_16/1, Scope16/1  "<testSig_CoETS_trqInrDesNTC>"
  BS_Result/16 -> cmp_16/2, Scope16/2  "<CoETS_trqInrDesNTC>"
  cmp_16/1 -> Bitwise_And16/1
  Bitwise_And16/1 -> AndN/16, Scope/16, tws_16/1

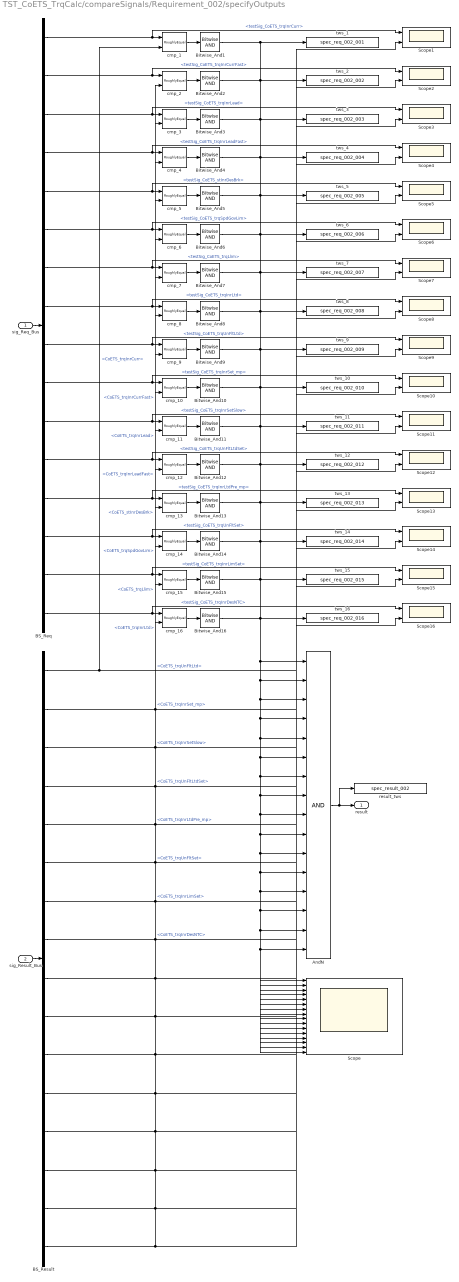
== system TST_CoETS_TrqCalc/compareSignals/Requirement_002/specifyOutputs ==
  sig_Req_Bus : Inport
  sig_Result_Bus : Inport  Port=2
  AndN : Logic  Inputs=16
  BS_Req : BusSelector  OutputSignals=testSig_CoETS_trqInrCurr,testSig_CoETS_trqInrCurrFast,testSig_CoETS_trqInrLead,testSig_CoETS_trqInrLeadFast,testSig_CoETS_stInrDesBrk,testSig_CoETS_trqSpdGovLim,testSig_CoETS_trqLlim,testSig_CoETS_trqInrLtd,testSig_CoETS_trqUnFltLtd,testSig_CoETS_trqInrSet_mp,testSig_CoETS_trqInrSetSlow,testSig_CoETS_trqUnFltLtdSet,testSig_CoETS_trqInrLtdPre_mp,testSig_CoETS_trqUnFltSet,testSig_CoETS_trqInrLimSet,testSig_CoETS_trqInrDesNTC
  BS_Result : BusSelector  OutputSignals=CoETS_trqInrCurr,CoETS_trqInrCurrFast,CoETS_trqInrLead,CoETS_trqInrLeadFast,CoETS_stInrDesBrk,CoETS_trqSpdGovLim,CoETS_trqLlim,CoETS_trqInrLtd,CoETS_trqUnFltLtd,CoETS_trqInrSet_mp,CoETS_trqInrSetSlow,CoETS_trqUnFltLtdSet,CoETS_trqInrLtdPre_mp,CoETS_trqUnFltSet,CoETS_trqInrLimSet,CoETS_trqInrDesNTC
  Bitwise_And{1..16} (16 alike) : simulink/Logic and Bit Operations/Bitwise Operator  logicop=AND  UseBitMask=off  BitMask=bin2dec('11011001')  BitMaskRealWorld=Stored Integer
  Scope : Scope  NumInputPorts=16
  Scope{1..16} (16 alike) : Scope  NumInputPorts=2
  cmp_{1..3,5..16} (15 alike) : UnitTest_Lib/RoughlyEqual  slope=0.1
  cmp_4 : UnitTest_Lib/RoughlyEqual  slope=0.5
  result_tws : ToWorkspace  VariableName=spec_result_002
  tws_1 : ToWorkspace  VariableName=spec_req_002_001
  tws_10 : ToWorkspace  VariableName=spec_req_002_010
  tws_11 : ToWorkspace  VariableName=spec_req_002_011
  tws_12 : ToWorkspace  VariableName=spec_req_002_012
  tws_13 : ToWorkspace  VariableName=spec_req_002_013
  tws_14 : ToWorkspace  VariableName=spec_req_002_014
  tws_15 : ToWorkspace  VariableName=spec_req_002_015
  tws_16 : ToWorkspace  VariableName=spec_req_002_016
  tws_2 : ToWorkspace  VariableName=spec_req_002_002
  tws_3 : ToWorkspace  VariableName=spec_req_002_003
  tws_4 : ToWorkspace  VariableName=spec_req_002_004
  tws_5 : ToWorkspace  VariableName=spec_req_002_005
  tws_6 : ToWorkspace  VariableName=spec_req_002_006
  tws_7 : ToWorkspace  VariableName=spec_req_002_007
  tws_8 : ToWorkspace  VariableName=spec_req_002_008
  tws_9 : ToWorkspace  VariableName=spec_req_002_009
  result : Outport
  wires:
  sig_Req_Bus/1 -> BS_Req/1
  sig_Result_Bus/1 -> BS_Result/1
  AndN/1 -> result/1, result_tws/1
  BS_Req/1 -> cmp_1/1, Scope1/1  "<testSig_CoETS_trqInrCurr>"
  BS_Result/1 -> cmp_1/2, Scope1/2  "<CoETS_trqInrCurr>"
  cmp_1/1 -> Bitwise_And1/1
  Bitwise_And1/1 -> AndN/1, Scope/1, tws_1/1
  BS_Req/2 -> cmp_2/1, Scope2/1  "<testSig_CoETS_trqInrCurrFast>"
  BS_Result/2 -> cmp_2/2, Scope2/2  "<CoETS_trqInrCurrFast>"
  cmp_2/1 -> Bitwise_And2/1
  Bitwise_And2/1 -> AndN/2, Scope/2, tws_2/1
  BS_Req/3 -> cmp_3/1, Scope3/1  "<testSig_CoETS_trqInrLead>"
  BS_Result/3 -> cmp_3/2, Scope3/2  "<CoETS_trqInrLead>"
  cmp_3/1 -> Bitwise_And3/1
  Bitwise_And3/1 -> AndN/3, Scope/3, tws_3/1
  BS_Req/4 -> cmp_4/1, Scope4/1  "<testSig_CoETS_trqInrLeadFast>"
  BS_Result/4 -> cmp_4/2, Scope4/2  "<CoETS_trqInrLeadFast>"
  cmp_4/1 -> Bitwise_And4/1
  Bitwise_And4/1 -> AndN/4, Scope/4, tws_4/1
  BS_Req/5 -> cmp_5/1, Scope5/1  "<testSig_CoETS_stInrDesBrk>"
  BS_Result/5 -> cmp_5/2, Scope5/2  "<CoETS_stInrDesBrk>"
  cmp_5/1 -> Bitwise_And5/1
  Bitwise_And5/1 -> AndN/5, Scope/5, tws_5/1
  BS_Req/6 -> cmp_6/1, Scope6/1  "<testSig_CoETS_trqSpdGovLim>"
  BS_Result/6 -> cmp_6/2, Scope6/2  "<CoETS_trqSpdGovLim>"
  cmp_6/1 -> Bitwise_And6/1
  Bitwise_And6/1 -> AndN/6, Scope/6, tws_6/1
  BS_Req/7 -> cmp_7/1, Scope7/1  "<testSig_CoETS_trqLlim>"
  BS_Result/7 -> cmp_7/2, Scope7/2  "<CoETS_trqLlim>"
  cmp_7/1 -> Bitwise_And7/1
  Bitwise_And7/1 -> AndN/7, Scope/7, tws_7/1
  BS_Req/8 -> cmp_8/1, Scope8/1  "<testSig_CoETS_trqInrLtd>"
  BS_Result/8 -> cmp_8/2, Scope8/2  "<CoETS_trqInrLtd>"
  cmp_8/1 -> Bitwise_And8/1
  Bitwise_And8/1 -> AndN/8, Scope/8, tws_8/1
  BS_Req/9 -> cmp_9/1, Scope9/1  "<testSig_CoETS_trqUnFltLtd>"
  BS_Result/9 -> cmp_9/2, Scope9/2  "<CoETS_trqUnFltLtd>"
  cmp_9/1 -> Bitwise_And9/1
  Bitwise_And9/1 -> AndN/9, Scope/9, tws_9/1
  BS_Req/10 -> cmp_10/1, Scope10/1  "<testSig_CoETS_trqInrSet_mp>"
  BS_Result/10 -> cmp_10/2, Scope10/2  "<CoETS_trqInrSet_mp>"
  cmp_10/1 -> Bitwise_And10/1
  Bitwise_And10/1 -> AndN/10, Scope/10, tws_10/1
  BS_Req/11 -> cmp_11/1, Scope11/1  "<testSig_CoETS_trqInrSetSlow>"
  BS_Result/11 -> cmp_11/2, Scope11/2  "<CoETS_trqInrSetSlow>"
  cmp_11/1 -> Bitwise_And11/1
  Bitwise_And11/1 -> AndN/11, Scope/11, tws_11/1
  BS_Req/12 -> cmp_12/1, Scope12/1  "<testSig_CoETS_trqUnFltLtdSet>"
  BS_Result/12 -> cmp_12/2, Scope12/2  "<CoETS_trqUnFltLtdSet>"
  cmp_12/1 -> Bitwise_And12/1
  Bitwise_And12/1 -> AndN/12, Scope/12, tws_12/1
  BS_Req/13 -> cmp_13/1, Scope13/1  "<testSig_CoETS_trqInrLtdPre_mp>"
  BS_Result/13 -> cmp_13/2, Scope13/2  "<CoETS_trqInrLtdPre_mp>"
  cmp_13/1 -> Bitwise_And13/1
  Bitwise_And13/1 -> AndN/13, Scope/13, tws_13/1
  BS_Req/14 -> cmp_14/1, Scope14/1  "<testSig_CoETS_trqUnFltSet>"
  BS_Result/14 -> cmp_14/2, Scope14/2  "<CoETS_trqUnFltSet>"
  cmp_14/1 -> Bitwise_And14/1
  Bitwise_And14/1 -> AndN/14, Scope/14, tws_14/1
  BS_Req/15 -> cmp_15/1, Scope15/1  "<testSig_CoETS_trqInrLimSet>"
  BS_Result/15 -> cmp_15/2, Scope15/2  "<CoETS_trqInrLimSet>"
  cmp_15/1 -> Bitwise_And15/1
  Bitwise_And15/1 -> AndN/15, Scope/15, tws_15/1
  BS_Req/16 -> cmp_16/1, Scope16/1  "<testSig_CoETS_trqInrDesNTC>"
  BS_Result/16 -> cmp_16/2, Scope16/2  "<CoETS_trqInrDesNTC>"
  cmp_16/1 -> Bitwise_And16/1
  Bitwise_And16/1 -> AndN/16, Scope/16, tws_16/1

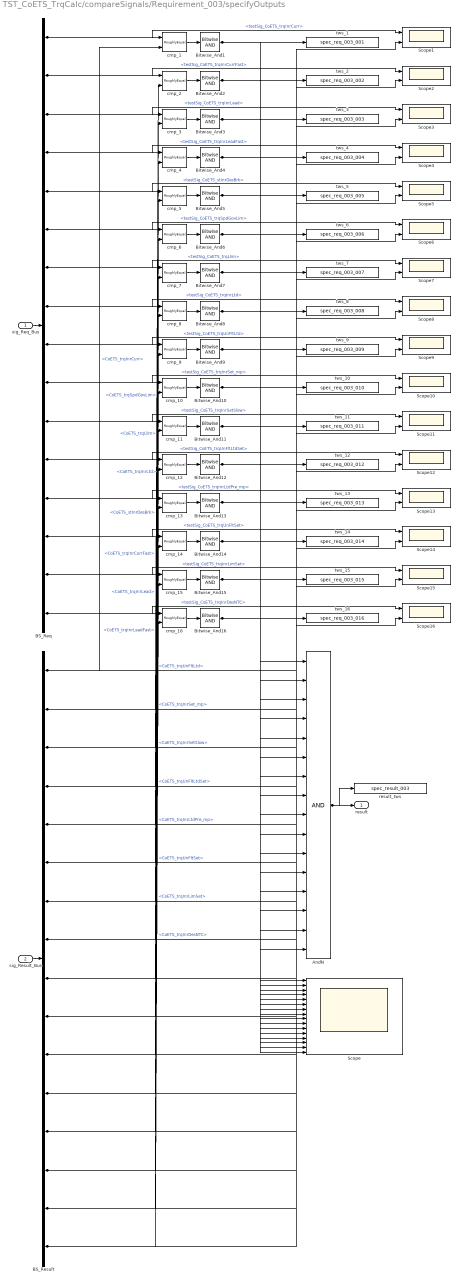
== system TST_CoETS_TrqCalc/compareSignals/Requirement_003/specifyOutputs ==
  sig_Req_Bus : Inport
  sig_Result_Bus : Inport  Port=2
  AndN : Logic  Inputs=16
  BS_Req : BusSelector  OutputSignals=testSig_CoETS_trqInrCurr,testSig_CoETS_trqInrCurrFast,testSig_CoETS_trqInrLead,testSig_CoETS_trqInrLeadFast,testSig_CoETS_stInrDesBrk,testSig_CoETS_trqSpdGovLim,testSig_CoETS_trqLlim,testSig_CoETS_trqInrLtd,testSig_CoETS_trqUnFltLtd,testSig_CoETS_trqInrSet_mp,testSig_CoETS_trqInrSetSlow,testSig_CoETS_trqUnFltLtdSet,testSig_CoETS_trqInrLtdPre_mp,testSig_CoETS_trqUnFltSet,testSig_CoETS_trqInrLimSet,testSig_CoETS_trqInrDesNTC
  BS_Result : BusSelector  OutputSignals=CoETS_trqInrCurr,CoETS_trqInrCurrFast,CoETS_trqInrLead,CoETS_trqInrLeadFast,CoETS_stInrDesBrk,CoETS_trqSpdGovLim,CoETS_trqLlim,CoETS_trqInrLtd,CoETS_trqUnFltLtd,CoETS_trqInrSet_mp,CoETS_trqInrSetSlow,CoETS_trqUnFltLtdSet,CoETS_trqInrLtdPre_mp,CoETS_trqUnFltSet,CoETS_trqInrLimSet,CoETS_trqInrDesNTC
  Bitwise_And{1..16} (16 alike) : simulink/Logic and Bit Operations/Bitwise Operator  logicop=AND  UseBitMask=off  BitMask=bin2dec('11011001')  BitMaskRealWorld=Stored Integer
  Scope : Scope  NumInputPorts=16
  Scope{1..16} (16 alike) : Scope  NumInputPorts=2
  cmp_{1..16} (16 alike) : UnitTest_Lib/RoughlyEqual  slope=0.1
  result_tws : ToWorkspace  VariableName=spec_result_003
  tws_1 : ToWorkspace  VariableName=spec_req_003_001
  tws_10 : ToWorkspace  VariableName=spec_req_003_010
  tws_11 : ToWorkspace  VariableName=spec_req_003_011
  tws_12 : ToWorkspace  VariableName=spec_req_003_012
  tws_13 : ToWorkspace  VariableName=spec_req_003_013
  tws_14 : ToWorkspace  VariableName=spec_req_003_014
  tws_15 : ToWorkspace  VariableName=spec_req_003_015
  tws_16 : ToWorkspace  VariableName=spec_req_003_016
  tws_2 : ToWorkspace  VariableName=spec_req_003_002
  tws_3 : ToWorkspace  VariableName=spec_req_003_003
  tws_4 : ToWorkspace  VariableName=spec_req_003_004
  tws_5 : ToWorkspace  VariableName=spec_req_003_005
  tws_6 : ToWorkspace  VariableName=spec_req_003_006
  tws_7 : ToWorkspace  VariableName=spec_req_003_007
  tws_8 : ToWorkspace  VariableName=spec_req_003_008
  tws_9 : ToWorkspace  VariableName=spec_req_003_009
  result : Outport
  wires:
  sig_Req_Bus/1 -> BS_Req/1
  sig_Result_Bus/1 -> BS_Result/1
  AndN/1 -> result/1, result_tws/1
  BS_Req/1 -> cmp_1/1, Scope1/1  "<testSig_CoETS_trqInrCurr>"
  BS_Result/1 -> cmp_1/2, Scope1/2  "<CoETS_trqInrCurr>"
  cmp_1/1 -> Bitwise_And1/1
  Bitwise_And1/1 -> tws_1/1, AndN/1, Scope/1
  BS_Req/2 -> cmp_2/1, Scope2/1  "<testSig_CoETS_trqInrCurrFast>"
  BS_Result/2 -> cmp_2/2, Scope2/2  "<CoETS_trqInrCurrFast>"
  cmp_2/1 -> Bitwise_And2/1
  Bitwise_And2/1 -> tws_2/1, AndN/2, Scope/2
  BS_Req/3 -> cmp_3/1, Scope3/1  "<testSig_CoETS_trqInrLead>"
  BS_Result/3 -> cmp_3/2, Scope3/2  "<CoETS_trqInrLead>"
  cmp_3/1 -> Bitwise_And3/1
  Bitwise_And3/1 -> tws_3/1, AndN/3, Scope/3
  BS_Req/4 -> cmp_4/1, Scope4/1  "<testSig_CoETS_trqInrLeadFast>"
  BS_Result/4 -> cmp_4/2, Scope4/2  "<CoETS_trqInrLeadFast>"
  cmp_4/1 -> Bitwise_And4/1
  Bitwise_And4/1 -> tws_4/1, AndN/4, Scope/4
  BS_Req/5 -> cmp_5/1, Scope5/1  "<testSig_CoETS_stInrDesBrk>"
  BS_Result/5 -> cmp_5/2, Scope5/2  "<CoETS_stInrDesBrk>"
  cmp_5/1 -> Bitwise_And5/1
  Bitwise_And5/1 -> tws_5/1, AndN/5, Scope/5
  BS_Req/6 -> cmp_6/1, Scope6/1  "<testSig_CoETS_trqSpdGovLim>"
  BS_Result/6 -> cmp_6/2, Scope6/2  "<CoETS_trqSpdGovLim>"
  cmp_6/1 -> Bitwise_And6/1
  Bitwise_And6/1 -> tws_6/1, AndN/6, Scope/6
  BS_Req/7 -> cmp_7/1, Scope7/1  "<testSig_CoETS_trqLlim>"
  BS_Result/7 -> cmp_7/2, Scope7/2  "<CoETS_trqLlim>"
  cmp_7/1 -> Bitwise_And7/1
  Bitwise_And7/1 -> tws_7/1, AndN/7, Scope/7
  BS_Req/8 -> cmp_8/1, Scope8/1  "<testSig_CoETS_trqInrLtd>"
  BS_Result/8 -> cmp_8/2, Scope8/2  "<CoETS_trqInrLtd>"
  cmp_8/1 -> Bitwise_And8/1
  Bitwise_And8/1 -> tws_8/1, AndN/8, Scope/8
  BS_Req/9 -> cmp_9/1, Scope9/1  "<testSig_CoETS_trqUnFltLtd>"
  BS_Result/9 -> cmp_9/2, Scope9/2  "<CoETS_trqUnFltLtd>"
  cmp_9/1 -> Bitwise_And9/1
  Bitwise_And9/1 -> tws_9/1, AndN/9, Scope/9
  BS_Req/10 -> cmp_10/1, Scope10/1  "<testSig_CoETS_trqInrSet_mp>"
  BS_Result/10 -> cmp_10/2, Scope10/2  "<CoETS_trqInrSet_mp>"
  cmp_10/1 -> Bitwise_And10/1
  Bitwise_And10/1 -> tws_10/1, AndN/10, Scope/10
  BS_Req/11 -> cmp_11/1, Scope11/1  "<testSig_CoETS_trqInrSetSlow>"
  BS_Result/11 -> cmp_11/2, Scope11/2  "<CoETS_trqInrSetSlow>"
  cmp_11/1 -> Bitwise_And11/1
  Bitwise_And11/1 -> tws_11/1, AndN/11, Scope/11
  BS_Req/12 -> cmp_12/1, Scope12/1  "<testSig_CoETS_trqUnFltLtdSet>"
  BS_Result/12 -> cmp_12/2, Scope12/2  "<CoETS_trqUnFltLtdSet>"
  cmp_12/1 -> Bitwise_And12/1
  Bitwise_And12/1 -> tws_12/1, AndN/12, Scope/12
  BS_Req/13 -> cmp_13/1, Scope13/1  "<testSig_CoETS_trqInrLtdPre_mp>"
  BS_Result/13 -> cmp_13/2, Scope13/2  "<CoETS_trqInrLtdPre_mp>"
  cmp_13/1 -> Bitwise_And13/1
  Bitwise_And13/1 -> tws_13/1, AndN/13, Scope/13
  BS_Req/14 -> cmp_14/1, Scope14/1  "<testSig_CoETS_trqUnFltSet>"
  BS_Result/14 -> cmp_14/2, Scope14/2  "<CoETS_trqUnFltSet>"
  cmp_14/1 -> Bitwise_And14/1
  Bitwise_And14/1 -> tws_14/1, AndN/14, Scope/14
  BS_Req/15 -> cmp_15/1, Scope15/1  "<testSig_CoETS_trqInrLimSet>"
  BS_Result/15 -> cmp_15/2, Scope15/2  "<CoETS_trqInrLimSet>"
  cmp_15/1 -> Bitwise_And15/1
  Bitwise_And15/1 -> tws_15/1, AndN/15, Scope/15
  BS_Req/16 -> cmp_16/1, Scope16/1  "<testSig_CoETS_trqInrDesNTC>"
  BS_Result/16 -> cmp_16/2, Scope16/2  "<CoETS_trqInrDesNTC>"
  cmp_16/1 -> Bitwise_And16/1
  Bitwise_And16/1 -> tws_16/1, AndN/16, Scope/16
